simulink model "subtract"  (R2020a)
settings: Solver=FixedStepAuto  StartTime=0.0  StopTime=10.0  RelTol=1e-3
PostLoadFcn:
  | config;
model workspace (MAT data in the model file):
  num1 = [10; 8]
  num2 = [2; 4]
  out = Simulink.SimulationOutput
  out.Data.logsout = Simulink.SimulationData.Dataset
  out.Data.logsout.any.Name = 'logsout'
  out.Data.logsout.any.Version = 3
  out.Data.logsout.any.Storage = Simulink.SimulationData.Storage.RamDatasetStorage
  out.Data.logsout.any.Storage.any.Version = 2
  out.Data.logsout.any.Storage.any.Elements{1} = Simulink.SimulationData.Signal
  out.Data.logsout.any.Storage.any.Elements{1}.PortType = 'outport'
  out.Data.logsout.any.Storage.any.Elements{1}.Version = 1
  out.Data.logsout.any.Storage.any.Elements{1}.BlockPath = Simulink.SimulationData.BlockPath
  out.Data.logsout.any.Storage.any.Elements{1}.BlockPath.path = {'subtract/Sum'}
  out.Data.logsout.any.Storage.any.Elements{1}.Values = timeseries
  out.Data.logsout.any.Storage.any.Elements{1}.Values.Name = 'out'
  out.Data.logsout.any.Storage.any.Elements{1}.Values.DataInfo = tsdata.datametadata
  out.Data.logsout.any.Storage.any.Elements{1}.Values.DataInfo.Interpolation = tsdata.interpolation
  out.Data.logsout.any.Storage.any.Elements{1}.Values.DataInfo.Interpolation.Fhandle : function handle (value not decoded)
  out.Data.logsout.any.Storage.any.Elements{1}.Values.DataInfo.Interpolation.Name = 'linear'
  out.Data.logsout.any.Storage.any.Elements{1}.Values.TimeInfo = tsdata.timemetadata
  out.Data.logsout.any.Storage.any.Elements{1}.Values.TimeInfo.Length = 51
  out.Data.logsout.any.Storage.any.Elements{1}.Values.TimeInfo.DuplicateTimes = 0
  out.Data.logsout.any.Storage.any.Elements{1}.Values.TimeInfo.Increment_ = 0.2
  out.Data.logsout.any.Storage.any.Elements{1}.Values.TimeInfo.Start_ = 0
  out.Data.logsout.any.Storage.any.Elements{1}.Values.TimeInfo.Initialized = 1
  out.Data.logsout.any.Storage.any.Elements{1}.Values.QualityInfo = tsdata.qualmetadata
  out.Data.logsout.any.Storage.any.Elements{1}.Values.Data_ = [6; 6; 6; 6; 6; 6; 6; 6; 6; 6; 6; 6; 6; 6; 6; 6; 6; 6; 6; 6; 6; 6; 6; 6; 6; 6; 6; 6; 6; 6; 6; 6; 6; 6; 6; 6; 6; 6; 6; 6; 6; 6; 6; 6; 6; 6; 6; 6; 6; 6; 6]
  out.Data.logsout.any.Storage.any.Elements{1}.Simulink.SimulationData.BlockData.VisualizationMetadata = Simulink.SimulationData.VisualizationMetadata
  out.Data.logsout.any.Storage.any.Elements{1}.Name = 'out'
  out.Data.tout = [0; 0.2; 0.4; 0.6; 0.8; 1; 1.2; 1.4; 1.6; 1.8; 2; 2.2; 2.4; 2.6; 2.8; 3; 3.2; 3.4; 3.6; 3.8; 4; 4.2; 4.4; 4.6; 4.8; 5; 5.2; 5.4; 5.6; 5.8; 6; 6.2; 6.4; 6.6; 6.8; 7; 7.2; 7.4; 7.6; 7.8; 8; 8.2; 8.4; 8.6; 8.8; 9; 9.2; 9.4; 9.6; 9.8; 10]
  out.Data.yout = Simulink.SimulationData.Dataset
  out.Data.yout.any.Name = 'yout'
  out.Data.yout.any.Version = 3
  out.Data.yout.any.Storage = Simulink.SimulationData.Storage.RamDatasetStorage
  out.Data.yout.any.Storage.any.Version = 2
  out.Data.yout.any.Storage.any.Elements{1} = Simulink.SimulationData.Signal
  out.Data.yout.any.Storage.any.Elements{1}.Version = 1
  out.Data.yout.any.Storage.any.Elements{1}.BlockPath = Simulink.SimulationData.BlockPath
  out.Data.yout.any.Storage.any.Elements{1}.BlockPath.path = {'subtract/Out1'}
  out.Data.yout.any.Storage.any.Elements{1}.Values = timeseries
  out.Data.yout.any.Storage.any.Elements{1}.Values.Name = 'Out1'
  out.Data.yout.any.Storage.any.Elements{1}.Values.DataInfo = tsdata.datametadata
  out.Data.yout.any.Storage.any.Elements{1}.Values.DataInfo.Interpolation = tsdata.interpolation
  out.Data.yout.any.Storage.any.Elements{1}.Values.DataInfo.Interpolation.Fhandle : function handle (value not decoded)
  out.Data.yout.any.Storage.any.Elements{1}.Values.DataInfo.Interpolation.Name = 'linear'
  out.Data.yout.any.Storage.any.Elements{1}.Values.TimeInfo = tsdata.timemetadata
  out.Data.yout.any.Storage.any.Elements{1}.Values.TimeInfo.Length = 51
  out.Data.yout.any.Storage.any.Elements{1}.Values.TimeInfo.DuplicateTimes = 0
  out.Data.yout.any.Storage.any.Elements{1}.Values.TimeInfo.Increment_ = 0.2
  out.Data.yout.any.Storage.any.Elements{1}.Values.TimeInfo.Start_ = 0
  out.Data.yout.any.Storage.any.Elements{1}.Values.TimeInfo.Initialized = 1
  out.Data.yout.any.Storage.any.Elements{1}.Values.QualityInfo = tsdata.qualmetadata
  out.Data.yout.any.Storage.any.Elements{1}.Values.Data_ = [6; 6; 6; 6; 6; 6; 6; 6; 6; 6; 6; 6; 6; 6; 6; 6; 6; 6; 6; 6; 6; 6; 6; 6; 6; 6; 6; 6; 6; 6; 6; 6; 6; 6; 6; 6; 6; 6; 6; 6; 6; 6; 6; 6; 6; 6; 6; 6; 6; 6; 6]
  out.Data.yout.any.Storage.any.Elements{1}.Simulink.SimulationData.BlockData.VisualizationMetadata = Simulink.SimulationData.VisualizationMetadata
  out.Data.yout.any.Storage.any.Elements{1}.Name = 'Out1'
  out.Metadata = Simulink.SimulationMetadata
  out.Metadata.ModelInfo.ModelName = 'subtract'
  out.Metadata.ModelInfo.ModelVersion = '1.11'
  out.Metadata.ModelInfo.ModelFilePath = 'D:\work\simulink_workspace\subtract_main\subtract.slx'
  out.Metadata.ModelInfo.UserID = 'P0158631'
  out.Metadata.ModelInfo.MachineName = 'INDDEV02'
  out.Metadata.ModelInfo.Platform = 'PCWIN64'
  out.Metadata.ModelInfo.ModelStructuralChecksum = [3425607607; 3314505699; 699772441; 1842305042]
  out.Metadata.ModelInfo.SimulationMode = 'normal'
  out.Metadata.ModelInfo.StartTime = 0
  out.Metadata.ModelInfo.StopTime = 10
  out.Metadata.ModelInfo.SolverInfo.Type = 'Fixed-Step'
  out.Metadata.ModelInfo.SolverInfo.Solver = 'FixedStepDiscrete'
  out.Metadata.ModelInfo.SolverInfo.FixedStepSize = 0.2
  out.Metadata.ModelInfo.SimulinkVersion.Name = 'Simulink'
  out.Metadata.ModelInfo.SimulinkVersion.Version = '10.1'
  out.Metadata.ModelInfo.SimulinkVersion.Release = '(R2020a)'
  out.Metadata.ModelInfo.SimulinkVersion.Date = '18-Nov-2019'
  out.Metadata.ModelInfo.LoggingInfo.LoggingToFile = 'off'
  out.Metadata.TimingInfo.WallClockTimestampStart = '2021-01-07 13:24:05'
  out.Metadata.TimingInfo.WallClockTimestampStop = '2021-01-07 13:24:11'
  out.Metadata.TimingInfo.InitializationElapsedWallTime = 4.3706531
  out.Metadata.TimingInfo.ExecutionElapsedWallTime = 0.8252111
  out.Metadata.TimingInfo.TerminationElapsedWallTime = 0.2494112
  out.Metadata.TimingInfo.TotalElapsedWallTime = 5.4452754
  out.Metadata.TimingInfo.ProfilerData = 'Profiler is not enabled'
  out.Metadata.ExecutionInfo.StopEvent = 'ReachedStopTime'
  out.Metadata.ExecutionInfo.StopEventSource = []
  out.Metadata.ExecutionInfo.StopEventDescription = 'Reached stop time of 10'
  out.Metadata.ExecutionInfo.ErrorDiagnostic = []
  out.Metadata.ExecutionInfo.WarningDiagnostics = struct([])
  out.Metadata.AppInfo = struct()
settings Model: OrderedModelArguments=off  Creator=P0158631  LastModifiedBy=P0158631
settings DataIOCC: ExternalInput=num1
settings OptimizationCC: ZeroExternalMemoryAtStartup=off  ZeroInternalMemoryAtStartup=off
settings DebuggingCC: UnderspecifiedInitializationDetection=Classic  MergeDetectMultiDrivingBlocksExec=none
settings ModelReferenceCC: PropagateSignalLabelsOutOfModel=off
settings RTWCC: Description=Generic Real-Time Target  GenCodeOnly=on  GenerateReport=on  LaunchReport=on  TargetLang=C++
settings GRTTargetCC: TargetLangStandard=C++03 (ISO)  MultiInstanceERTCode=on  CodeInterfacePackaging=C++ class

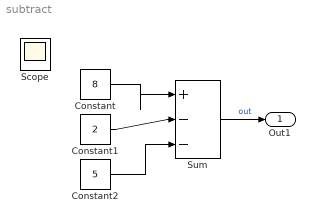
== system subtract ==
  Constant : Constant  Value=8
  Constant1 : Constant  Value=2
  Constant2 : Constant  Value=5
  Sum : Sum  Inputs=|+--
  Out1 : Outport  SignalName=Out1
  Scope : Scope
  wires:
  Sum/1 -> Out1/1  "out"
  Constant/1 -> Sum/1
  Constant1/1 -> Sum/2
  Constant2/1 -> Sum/3
